simulink model "quad_copter_model"  (R2016a)
settings: Solver=VariableStepAuto  StartTime=0.0  StopTime=70  RelTol=1e-3
values from neighbouring files (symbols this model uses):
  Mixer = tf(66.6667,      'InputName', 'dM', 'OutputName', 'd\Omega')    [mk_quad_copter_models.m]    (also in slx_data.m = 66.6666666667)
  PitchRateModel_tf = tf(PitchRateModel)    [slx_data.m]
  R1 = pid(.3, .3, .05, Tf)    [slx_data.m]
  R2 = pid(1.61, 0, .00512, Tf)    [slx_data.m]
  step_size = .18    (= 0.18)    [mk_quad_copter_models.m]
libraries: simulink x2
settings Model: Creator=tibo  LastModifiedBy=tibo

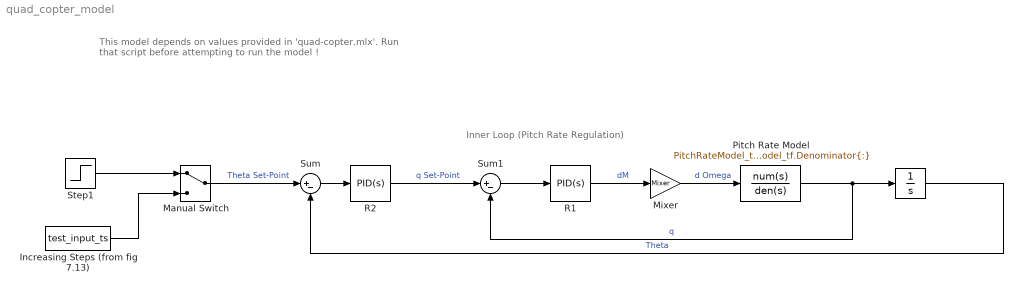
== system quad_copter_model ==
  note: Inner Loop (Pitch Rate Regulation)
  note: This model depends on values provided in 'quad-copter.mlx'.
      | Run that script before attempting to run the model !
  " " : Integrator  ContinuousStateAttributes='PitchAngle'
  Increasing Steps (from fig 7.13) : FromWorkspace  VariableName=test_input_ts  SampleTime=0  OutputAfterFinalValue=Holding final value
  Manual Switch : ManualSwitch
  "Mixer " : Gain  Gain=Mixer
  "Pitch Rate Model " : TransferFcn  Numerator=PitchRateModel_tf.Numerator{:}  Denominator=PitchRateModel_tf.Denominator{:}  ContinuousStateAttributes='PitchRate'
  "R1 " : simulink/Continuous/PID Controller  Controller=PID  TimeDomain=Continuous-time  SampleTime=-1  IntegratorMethod=Forward Euler  FilterMethod=Forward Euler  Form=Parallel  UseFilter=on  ControllerParametersSource=internal  P=R1.Kp  I=R1.Ki  D=R1.Kd  N=R1.Tf  InitialConditionSource=internal  InitialConditionForIntegrator=0  InitialConditionForFilter=0  ExternalReset=none  LimitOutput=off  UpperSaturationLimit=inf  LowerSaturationLimit=-inf  LinearizeAsGain=on  AntiWindupMode=none  Kb=1  TrackingMode=off  Kt=1  PParamMin=[]  PParamMax=[]  IParamMin=[]  IParamMax=[]  DParamMin=[]  DParamMax=[]  NParamMin=[]  NParamMax=[]  KbParamMin=[]  KbParamMax=[]  KtParamMin=[]  KtParamMax=[]  POutMin=[]  POutMax=[]  IOutMin=[]  IOutMax=[]  DOutMin=[]  DOutMax=[]  NOutMin=[]  NOutMax=[]  KbOutMin=[]  KbOutMax=[]  KtOutMin=[]  KtOutMax=[]  IntegratorOutMin=[]  IntegratorOutMax=[]  FilterOutMin=[]  FilterOutMax=[]  SumOutMin=[]  SumOutMax=[]  SumI1OutMin=[]  SumI1OutMax=[]  SumI2OutMin=[]  SumI2OutMax=[]  SumI3OutMin=[]  SumI3OutMax=[]  SumDOutMin=[]  SumDOutMax=[]  SaturationOutMin=[]  SaturationOutMax=[]  IntegratorContinuousStateAttributes=''  IntegratorStateMustResolveToSignalObject=off  IntegratorRTWStateStorageClass=Auto  FilterContinuousStateAttributes=''  FilterStateMustResolveToSignalObject=off  FilterRTWStateStorageClass=Auto  DifferentiatorICPrevScaledInput=0  DifferentiatorOutMin=[]  DifferentiatorOutMax=[]
  "R2 " : simulink/Continuous/PID Controller  Controller=PID  TimeDomain=Continuous-time  SampleTime=-1  IntegratorMethod=Forward Euler  FilterMethod=Forward Euler  Form=Parallel  UseFilter=on  ControllerParametersSource=internal  P=R2.Kp  I=R2.Ki  D=R2.Kd  N=R2.Tf  InitialConditionSource=internal  InitialConditionForIntegrator=0  InitialConditionForFilter=0  ExternalReset=none  LimitOutput=off  UpperSaturationLimit=inf  LowerSaturationLimit=-inf  LinearizeAsGain=on  AntiWindupMode=none  Kb=1  TrackingMode=off  Kt=1  PParamMin=[]  PParamMax=[]  IParamMin=[]  IParamMax=[]  DParamMin=[]  DParamMax=[]  NParamMin=[]  NParamMax=[]  KbParamMin=[]  KbParamMax=[]  KtParamMin=[]  KtParamMax=[]  POutMin=[]  POutMax=[]  IOutMin=[]  IOutMax=[]  DOutMin=[]  DOutMax=[]  NOutMin=[]  NOutMax=[]  KbOutMin=[]  KbOutMax=[]  KtOutMin=[]  KtOutMax=[]  IntegratorOutMin=[]  IntegratorOutMax=[]  FilterOutMin=[]  FilterOutMax=[]  SumOutMin=[]  SumOutMax=[]  SumI1OutMin=[]  SumI1OutMax=[]  SumI2OutMin=[]  SumI2OutMax=[]  SumI3OutMin=[]  SumI3OutMax=[]  SumDOutMin=[]  SumDOutMax=[]  SaturationOutMin=[]  SaturationOutMax=[]  IntegratorContinuousStateAttributes=''  IntegratorStateMustResolveToSignalObject=off  IntegratorRTWStateStorageClass=Auto  FilterContinuousStateAttributes=''  FilterStateMustResolveToSignalObject=off  FilterRTWStateStorageClass=Auto  DifferentiatorICPrevScaledInput=0  DifferentiatorOutMin=[]  DifferentiatorOutMax=[]
  Step1 : Step  After=step_size  SampleTime=0
  Sum : Sum  Inputs=|+-
  Sum1 : Sum  Inputs=|+-
  wires:
  Manual Switch/1 -> Sum/1  "Theta Set-Point"
  Sum/1 -> "R2 "/1
  "R2 "/1 -> Sum1/1  "q Set-Point"
  Sum1/1 -> "R1 "/1
  "R1 "/1 -> "Mixer "/1  "dM"
  "Mixer "/1 -> "Pitch Rate Model "/1  "d Omega"
  "Pitch Rate Model "/1 -> Sum1/2, " "/1  "q"
  " "/1 -> Sum/2  "Theta"
  Increasing Steps (from fig 7.13)/1 -> Manual Switch/2
  Step1/1 -> Manual Switch/1
